simulink model "mm5"  (R2024a)
settings: Solver=VariableStepAuto  StartTime=0.0  StopTime=30  RelTol=1e-3
model workspace (MAT data in the model file):
  n = Simulink.Parameter
  n.Complexity = 'real'
  n.Dimensions = [0 0]
  n.DataType = 'auto'
values from neighbouring files (symbols this model uses):
  n = 10    [arima_forecast.m]    (also in queue_sim.m = 5)
undefined symbols (not defined in the file or in its folder): m, pause
settings Model: Creator=amarn  LastModifiedBy=amarn

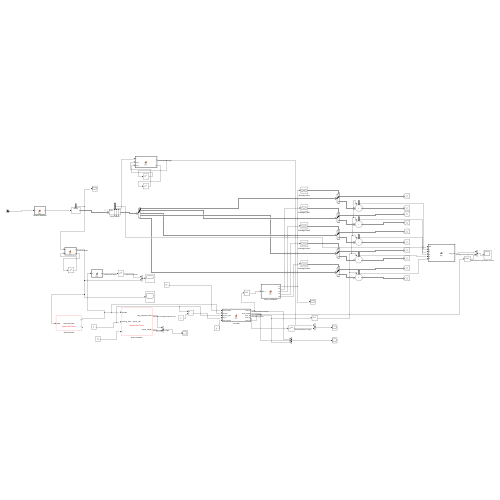
[thumbnail: Simulink's stored preview of the top-level diagram]
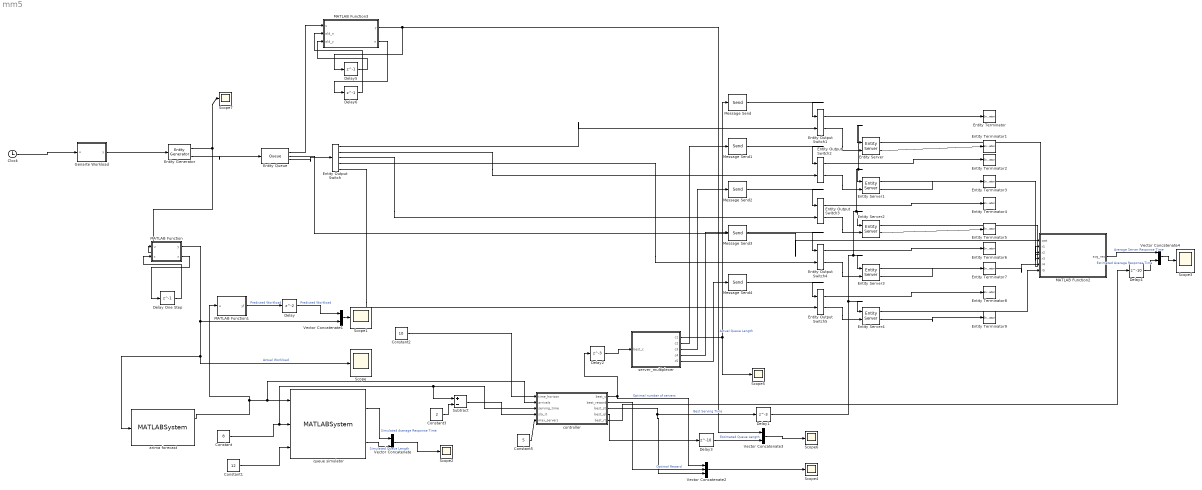
== system mm5 ==
  Clock : Clock
  Constant : Constant  Value=8
  Constant1 : Constant  Value=12
  Constant2 : Constant  Value=10
  Constant3 : Constant  Value=2
  Constant5 : Constant  Value=5
  Delay : Delay
  Delay One Step : Delay  DelayLength=1
  Delay1 : Delay  DelayLength=3
  Delay2 : Delay  DelayLength=3
  Delay3 : Delay  DelayLength=10
  Delay4 : Delay  DelayLength=10
  Delay5 : Delay  DelayLength=1
  Delay6 : Delay  DelayLength=1
  Entity Output Switch : EntityOutputSwitch  InputPortMessageModes=m  OutputPortMessageModes=m,m,m,m,m  NumberOutputPorts=5  SwitchAttributeName=Attribute1
      settings: OutputPortMap=o0,o1,o2,o3,o4
  Entity Output Switch1 : EntityOutputSwitch  InputPortMessageModes=m,m  OutputPortMessageModes=m,m  SwitchingCriterion=From control port  SwitchAttributeName=Attribute1  InitialPortSelection=2
      settings: InputPortMap=u0,u1
  Entity Output Switch2 : EntityOutputSwitch  InputPortMessageModes=m,m  OutputPortMessageModes=m,m  SwitchingCriterion=From control port  SwitchAttributeName=Attribute1  InitialPortSelection=2
      settings: InputPortMap=u0,u1
  Entity Output Switch3 : EntityOutputSwitch  InputPortMessageModes=m,m  OutputPortMessageModes=m,m  SwitchingCriterion=From control port  SwitchAttributeName=Attribute1
      settings: InputPortMap=u0,u1
  Entity Output Switch4 : EntityOutputSwitch  InputPortMessageModes=m,m  OutputPortMessageModes=m,m  SwitchingCriterion=From control port  SwitchAttributeName=Attribute1
      settings: InputPortMap=u0,u1
  Entity Output Switch5 : EntityOutputSwitch  InputPortMessageModes=m,m  OutputPortMessageModes=m,m  SwitchingCriterion=From control port  SwitchAttributeName=Attribute1
      settings: InputPortMap=u0,u1
  Entity Generator : EntityGenerator  OutputPortMessageModes=n,m  TimeSource=Signal port  IntergenerationTimeAction=|  NumberEntitiesDeparted=on  EntityType=Structured  EntityTypeName=Entity
      | % Pattern: Exponential distribution
      | mu = 0.3;
      | x1 = -mu * log(1 - rand());
      | dt=x1;
      settings: InputPortMap=u1  OutputPortMap=o0,o3
  Entity Queue : Queue  InputPortMessageModes=m  OutputPortMessageModes=n,n,m  Capacity=Inf  EntryAction=pause(4);  NumberEntitiesInBlock=on  AverageWait=on
      settings: OutputPortMap=o1,o2,o5
  Entity Server{,1..4} (5 alike) : EntityServer  InputPortMessageModes=n,m  OutputPortMessageModes=n,m  Capacity=1  ServiceTimeSource=Signal port  Utilization=on
      settings: InputPortMap=u0,u2  OutputPortMap=o5,o9
  Entity Terminator{,1..9} (10 alike) : EntityTerminator  InputPortMessageModes=m
  Genarte Workload : MATLAB Function  TreatAsAtomicUnit=on
  MATLAB Function : MATLAB Function  TreatAsAtomicUnit=on
  MATLAB Function1 : MATLAB Function  TreatAsAtomicUnit=on
  MATLAB Function2 : MATLAB Function  TreatAsAtomicUnit=on
  MATLAB Function3 : MATLAB Function  TreatAsAtomicUnit=on
  Message Send{,1..4} (5 alike) : Send  OutputPortMessageModes=m
  Scope{,1..7} (8 alike) : Scope
  Subtract : Sum  Inputs=+-
  Vector Concatenate{,1,3..4} (4 alike) : Concatenate
  Vector Concatenate2 : Concatenate  NumInputs=3
  arima forecast : MATLABSystem  System=arima_forecast  n=10  p=1  q=1  D=1  SimulateUsing=Interpreted execution
      mask Type: arima_forecast
      mask Display:
      | disp('arima_forecast');
      | port_label('input',1,'ynew');
      | port_label('output',1,'y');
      | port_label('output',2,'t');
  controller : MATLAB Function  TreatAsAtomicUnit=on
  queue simulator : MATLABSystem  System=queue_sim  time_horizon=int32(10)  n=5  res=0  SimulateUsing=Interpreted execution
      mask Type: queue_sim
      mask Display:
      | disp('queue_sim');
      | port_label('input',1,'arrivals');
      | port_label('input',2,'serving_time');
      | port_label('input',3,'c');
      | port_label('output',1,'avg_response_time');
      | port_label('output',2,'queue_length');
  server_multiplexer : MATLAB Function  TreatAsAtomicUnit=on
  wires:
  Entity Generator/2 -> Entity Queue/1
  Entity Queue/3 -> Entity Output Switch/1
  Entity Output Switch1/1 -> Entity Terminator/1
  Entity Output Switch2/1 -> Entity Terminator2/1
  Entity Output Switch3/1 -> Entity Terminator4/1
  Entity Output Switch4/1 -> Entity Terminator6/1
  Entity Output Switch5/1 -> Entity Terminator8/1
  Entity Output Switch/1 -> Entity Output Switch1/2
  Entity Output Switch/2 -> Entity Output Switch2/2
  Entity Output Switch/3 -> Entity Output Switch3/2
  Entity Output Switch/4 -> Entity Output Switch4/2
  Entity Output Switch/5 -> Entity Output Switch5/2
  Entity Output Switch1/2 -> Entity Server/2
  Entity Server/2 -> Entity Terminator1/1
  Entity Output Switch2/2 -> Entity Server1/2
  Entity Server1/2 -> Entity Terminator3/1
  Entity Output Switch3/2 -> Entity Server2/2
  Entity Server2/2 -> Entity Terminator5/1
  Entity Output Switch4/2 -> Entity Server3/2
  Entity Server3/2 -> Entity Terminator7/1
  Entity Output Switch5/2 -> Entity Server4/2
  Entity Server4/2 -> Entity Terminator9/1
  Entity Generator/1 -> MATLAB Function/1(u), Scope7/1
  MATLAB Function/1(y) -> Scope/1, arima forecast/1, Vector Concatenate1/2  "Actual Workload"
  MATLAB Function/2(x) -> Delay One Step/1
  Delay One Step/1 -> MATLAB Function/2("x ")
  arima forecast/1 -> MATLAB Function1/1(u), controller/2(arrivals), queue simulator/1
  Vector Concatenate1/1 -> Scope1/1
  Constant/1 -> Subtract/1, controller/3(serving_time), queue simulator/2
  queue simulator/1 -> Vector Concatenate/1  "Simulated Average Response Time"
  queue simulator/2 -> Vector Concatenate/2  "Simulated Queue Length"
  Vector Concatenate/1 -> Scope2/1
  Constant1/1 -> queue simulator/3
  Constant2/1 -> controller/1(time_horizon)
  controller/1(best_c) -> Vector Concatenate2/1, Delay2/1  "Optimal number of servers"
  controller/2(best_reward) -> Vector Concatenate2/2  "Optimal Reward"
  Vector Concatenate2/1 -> Scope4/1
  Message Send/1 -> Entity Output Switch1/1
  server_multiplexer/2(c2) -> Message Send1/1
  Message Send1/1 -> Entity Output Switch2/1
  server_multiplexer/3(c3) -> Message Send2/1
  Message Send2/1 -> Entity Output Switch3/1
  server_multiplexer/4(c4) -> Message Send3/1
  Message Send3/1 -> Entity Output Switch4/1
  server_multiplexer/5(c5) -> Message Send4/1
  Message Send4/1 -> Entity Output Switch5/1
  server_multiplexer/1(c1) -> Scope5/1, Message Send/1
  Entity Queue/2 -> MATLAB Function2/1(qwt)
  Entity Server/1 -> MATLAB Function2/2(r1)
  Entity Server1/1 -> MATLAB Function2/3(r2)
  Entity Server2/1 -> MATLAB Function2/4(r3)
  Entity Server3/1 -> MATLAB Function2/5(r4)
  Entity Server4/1 -> MATLAB Function2/6(r5)
  MATLAB Function1/1(yf) -> Delay/1  "Predicted Workload"
  Delay/1 -> Vector Concatenate1/1  "Predicted Workload"
  Constant3/1 -> Subtract/2
  Subtract/1 -> controller/4(sla_rt)
  controller/3(best_st) -> Vector Concatenate2/3, Delay1/1  "Best Serving Time"
  Constant5/1 -> controller/5(max_servers)
  Delay1/1 -> Entity Server/1, Entity Server1/1, Entity Server2/1, Entity Server3/1, Entity Server4/1
  Delay2/1 -> server_multiplexer/1(best_c)
  controller/4(best_ql) -> Delay3/1
  Delay3/1 -> Vector Concatenate3/2  "Estimated Queue Length"
  Vector Concatenate3/1 -> Scope6/1
  MATLAB Function2/1(avg_res) -> Vector Concatenate4/1  "Average Server Response Time"
  Vector Concatenate4/1 -> Scope3/1
  Delay4/1 -> Vector Concatenate4/2  "Estimated Average Response Time"
  controller/5(best_rt) -> Delay4/1
  MATLAB Function3/1(y) -> Delay5/1, Vector Concatenate3/1  "Actual Queue Length"
  Entity Queue/1 -> MATLAB Function3/1(u)
  Delay5/1 -> MATLAB Function3/3(old_y)
  MATLAB Function3/2(n) -> Delay6/1
  Delay6/1 -> MATLAB Function3/2(old_n)
  Clock/1 -> Genarte Workload/1(u)
  Genarte Workload/1(y) -> Entity Generator/1

== matlab function mm5/MATLAB Function1 ==
  data: u input; yf output
function yf = fcn(u)

yf = u(1);

== matlab function mm5/MATLAB Function ==
  data: u input; y output; x input; x output
function [y, x] = fcn(u, x)
y=u-x;
x=u;

== matlab function mm5/controller ==
  data: time_horizon input; best_c output; arrivals input; serving_time input; best_reward output; sla_rt input; best_st output; max_servers input; best_ql output; best_rt output
function [best_c,best_reward,best_st,best_ql,best_rt] = fcn(time_horizon,arrivals,serving_time,sla_rt,max_servers)
max_c=-1;
max_reward=-10000;
%min_st=serving_time;
st=serving_time;
min_st=st;
min_rt=-1;
min_ql=-1;
for c= (1:max_servers)
    [avg_response_time,queue_length]=controller(time_horizon,arrivals,st,c);
    sla_gain=0;
    e_consumption=0.5*(c)/(max_servers);
    if avg_response_time<=sla_rt
        sla_gain=1;
        %figure out a way to increase rt
        %st=round(st*(1+c/max_servers));we haven't put an incentive to have higher as compared to lower c
    else
        sla_gain=-1;
        st=round(st*(1-c/max_servers));
        min_st=st;
    end
    reward=sla_gain-e_consumption;
    disp('Reward for');
    disp(c);
    disp('is : ');
    disp(reward);
    disp('Serving time is :');
    disp(st);
    if reward>max_reward
       max_c=c;
       max_reward=reward;
       min_rt=avg_response_time;
       min_ql=queue_length;
    end
    %disp('For:');
    %disp(c);
    disp('Best reward is :');
    disp(max_reward);
    disp('Best c is :');
    disp(max_c);
end
best_c=max_c;
best_reward=max_reward;
best_st=min_st;
best_rt=min_rt;
best_ql=min_ql;
end

== matlab function mm5/server_multiplexer ==
  data: best_c input; c1 output; c2 output; c3 output; c4 output; c5 output
function [c1,c2,c3,c4,c5] = fcn(best_c)
    c1=1;
    c2=1;
    c3=1;
    c4=1;
    c5=1;
    temp=ones(5,1);
    for i =(1:best_c)
        temp(i)=2;
    end
    if best_c==1
        c1=2;
    end
    if best_c==2
        c1=2;
        c2=2;
    end
    if best_c==3
        c1=2;
        c2=2;
        c3=2;
    end
    if best_c==4
        c1=2;
        c2=2;
        c3=2;
        c4=2;
    end
    if best_c==4
        c1=2;
        c2=2;
        c3=2;
        c4=2;
        c5=2;
    end
    %t = num2cell(temp);
    %[c1,c2,c3,c4,c5]=t{:};
end

== matlab function mm5/MATLAB Function2 ==
  data: qwt input; r1 input; avg_res output; r2 input; r3 input; r4 input; r5 input
function avg_res = fcn(qwt,r1,r2,r3,r4,r5)
    avg_res=(r1+r2+r3+r4+r5)*30/5+qwt;
end

== matlab function mm5/MATLAB Function3 ==
  data: u input; y output; old_n input; n output; old_y input
function [y,n] = fcn(u,old_n,old_y)
n=old_n+1;
%sum_u=sum(list_u)+u;
avg_u=(old_n*old_y+u)/n;
y = avg_u;

== matlab function mm5/Genarte Workload ==
  data: u input; y output
function y = fcn(u)
    
y = 3*(1-u/30);
